simulink model "cannon2_group03"  (R2021a)
settings: Solver=VariableStepAuto  StartTime=0.0  StopTime=20  RelTol=1e-3
settings Model: Creator=zeoliam  LastModifiedBy=zeoliam

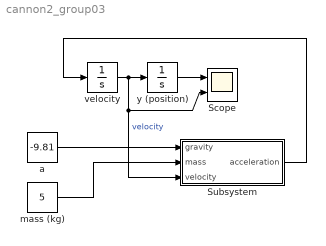
== system cannon2_group03 ==
  Scope : Scope  NumInputPorts=2
  Subsystem : Subsystem
  a : Constant  Value=-9.81
  mass (kg) : Constant  Value=5
  velocity : Integrator
  y (position) : Integrator
  wires:
  mass (kg)/1 -> Subsystem/2(mass)
  velocity/1 -> Subsystem/3(velocity), Scope/2, y (position)/1  "velocity"
  y (position)/1 -> Scope/1
  a/1 -> Subsystem/1(gravity)
  Subsystem/1(acceleration) -> velocity/1

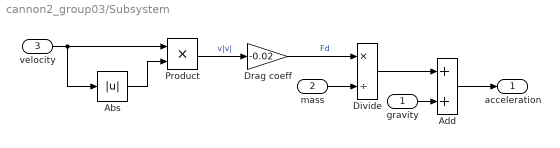
== system cannon2_group03/Subsystem ==
  gravity : Inport
  mass : Inport  Port=2
  velocity : Inport  Port=3
  Abs : Abs
  Add : Sum
  Divide : Product  Inputs=*/
  Drag coeff : Gain  Gain=-0.02
  Product : Product
  acceleration : Outport
  wires:
  velocity/1 -> Abs/1, Product/1
  Abs/1 -> Product/2
  Product/1 -> Drag coeff/1  "v|v|"
  Drag coeff/1 -> Divide/1  "Fd"
  mass/1 -> Divide/2
  Divide/1 -> Add/1
  gravity/1 -> Add/2
  Add/1 -> acceleration/1
